simulink model "ARDronePFC"  (R2023b)
settings: Solver=ode1  StartTime=0.0  StopTime=200  FixedStep=simDT  RelTol=1e-3  EnableMultiTasking=on
values from neighbouring files (symbols this model uses):
  timeDelay = FMS.Ts*4    [setupEPFC.m]    (also in setupPFC.m)
undefined symbols (not defined in the file or in its folder): ssH, ssPitch, ssPitch2U, ssRoll, ssRoll2V, ssYaw
libraries: ARBlocks x3

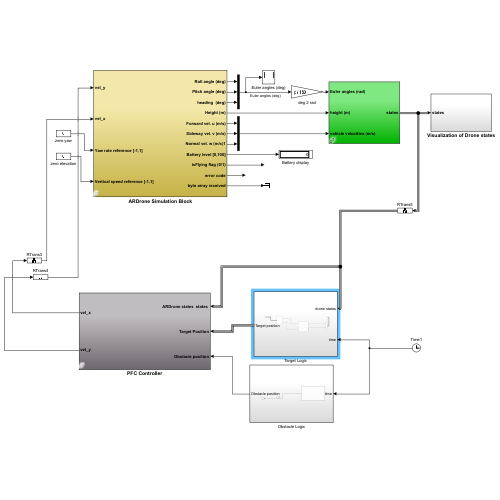
[thumbnail: Simulink's stored preview of the top-level diagram]
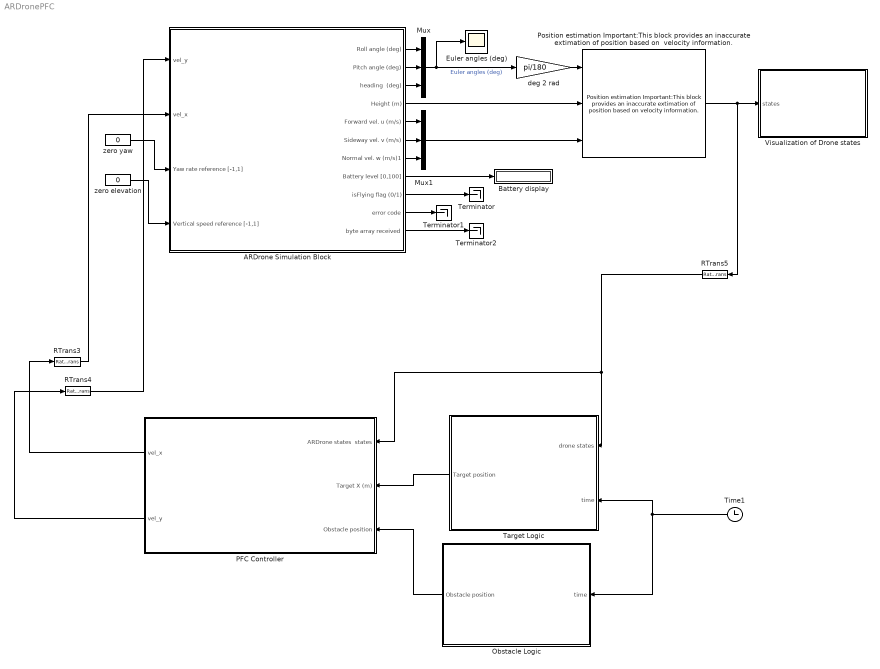
== system ARDronePFC ==
  ARDrone Simulation Block : Subsystem  AncestorBlock=ARBlocks/ARDrone Simulation Block
  Battery display : Display
  Euler angles (deg) : Scope
  Mux : Mux  Inputs=3
  Mux1 : Mux  Inputs=3
  Obstacle Logic : Subsystem
  PFC Controller : Subsystem  AncestorBlock=ARBlocks/Baseline Controller
  "Position estimation Important:This block provides an inaccurate extimation of position based on  velocity information. " : ARBlocks/Position estimation Important:This block provides an  inaccurate extimation of position  based on  velocity information.   SystemSampleTime=-1  VariantActivationTime=update diagram  AllowFlexibleInterface=on  Latency=0  AutoFrameSizeCalculation=off
  RTrans3 : RateTransition  OutPortSampleTime=simDT
  RTrans4 : RateTransition  OutPortSampleTime=simDT
  RTrans5 : RateTransition  OutPortSampleTime=FMS.Ts
  Target Logic : Subsystem
  Terminator : Terminator
  Terminator1 : Terminator
  Terminator2 : Terminator
  Time1 : Clock
  Visualization of Drone states : Subsystem
  deg 2 rad : Gain  Gain=pi/180
  zero elevation : Constant  Value=0
  zero yaw : Constant  Value=0
  wires:
  ARDrone Simulation Block/1(Roll angle (deg)) -> Mux/1
  ARDrone Simulation Block/2(Pitch angle (deg)) -> Mux/2
  ARDrone Simulation Block/5(Forward vel. u (m/s)) -> Mux1/1
  ARDrone Simulation Block/6(Sideway vel. v (m/s)) -> Mux1/2
  ARDrone Simulation Block/7(Normal vel. w (m/s)1) -> Mux1/3
  Mux/1 -> deg 2 rad/1, Euler angles (deg)/1  "Euler angles (deg)"
  ARDrone Simulation Block/8(Battery level [0,100]) -> Battery display/1
  PFC Controller/1(vel_x) -> RTrans3/1
  "Position estimation Important:This block provides an inaccurate extimation of position based on  velocity information. "/1 -> RTrans5/1, Visualization of Drone states/1(states)
  deg 2 rad/1 -> "Position estimation Important:This block provides an inaccurate extimation of position based on  velocity information. "/1
  ARDrone Simulation Block/4(Height (m)) -> "Position estimation Important:This block provides an inaccurate extimation of position based on  velocity information. "/2
  Mux1/1 -> "Position estimation Important:This block provides an inaccurate extimation of position based on  velocity information. "/3
  PFC Controller/2(vel_y) -> RTrans4/1
  ARDrone Simulation Block/3(heading  (deg)) -> Mux/3
  ARDrone Simulation Block/9(isFlying flag (0/1)) -> Terminator/1
  RTrans3/1 -> ARDrone Simulation Block/2(vel_x)
  RTrans4/1 -> ARDrone Simulation Block/1(vel_y)
  ARDrone Simulation Block/10(error code) -> Terminator1/1
  ARDrone Simulation Block/11(byte array received) -> Terminator2/1
  RTrans5/1 -> Target Logic/1(drone states), PFC Controller/1("ARDrone states  states ")
  zero yaw/1 -> ARDrone Simulation Block/3(Yaw rate reference [-1,1])
  zero elevation/1 -> ARDrone Simulation Block/4(Vertical speed reference [-1,1])
  Target Logic/1(Target position) -> PFC Controller/2(Target X (m))
  Obstacle Logic/1(Obstacle position) -> PFC Controller/3(Obstacle position)
  Time1/1 -> Target Logic/2(time), Obstacle Logic/1(time)

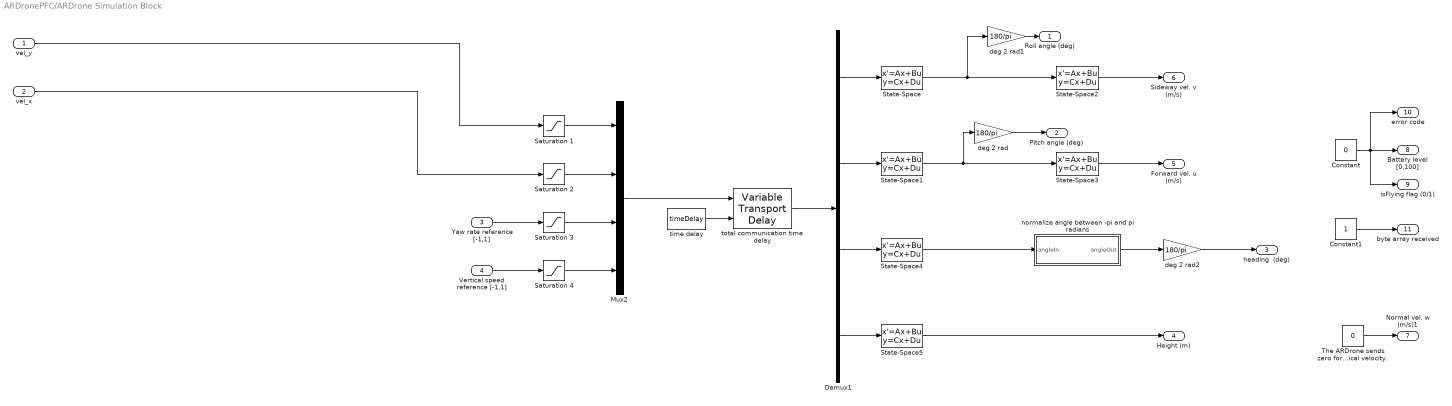
== system ARDronePFC/ARDrone Simulation Block ==
  vel_y : Inport
  vel_x : Inport  Port=2
  Yaw rate reference [-1,1] : Inport  Port=3
  Vertical speed reference [-1,1] : Inport  Port=4
  Constant : Constant  Value=0
  Constant1 : Constant
  Demux1 : Demux
  Mux2 : Mux
  Saturation {1..4} (4 alike) : Saturate  UpperLimit=1  LowerLimit=-1
  State-Space : StateSpace  A=ssRoll.a  B=ssRoll.b  C=ssRoll.c  D=ssRoll.d  InitialCondition=0
  State-Space1 : StateSpace  A=ssPitch.a  B=ssPitch.b  C=ssPitch.c  D=ssPitch.d  InitialCondition=0
  State-Space2 : StateSpace  A=ssRoll2V.a  B=ssRoll2V.b  C=ssRoll2V.c  D=ssRoll2V.d  InitialCondition=0
  State-Space3 : StateSpace  A=ssPitch2U.a  B=ssPitch2U.b  C=ssPitch2U.c  D=ssPitch2U.d  InitialCondition=0
  State-Space4 : StateSpace  A=ssYaw.a  B=ssYaw.b  C=ssYaw.c  D=ssYaw.d  InitialCondition=0
  State-Space5 : StateSpace  A=ssH.a  B=ssH.b  C=ssH.c  D=ssH.d  InitialCondition=0
  "The ARDrone sends zero for the vertical velocity. " : Constant  Value=0
  deg 2 rad : Gain  Gain=180/pi
  deg 2 rad1 : Gain  Gain=180/pi
  deg 2 rad2 : Gain  Gain=180/pi
  normalize angle between -pi and pi radians : MATLAB Function  TreatAsAtomicUnit=on
  time delay : Constant  Value=timeDelay
  total communication time delay : VariableTransportDelay  MaximumDelay=10  InitialOutput=[0 0 0 0]  MaximumPoints=4096
  Roll angle (deg) : Outport
  Pitch angle (deg) : Outport  Port=2
  heading  (deg) : Outport  Port=3
  Height (m) : Outport  Port=4
  Forward vel. u (m/s) : Outport  Port=5
  Sideway vel. v (m/s) : Outport  Port=6
  Normal vel. w (m/s)1 : Outport  Port=7
  Battery level [0,100] : Outport  Port=8
  isFlying flag (0/1) : Outport  Port=9
  error code : Outport  Port=10
  byte array received : Outport  Port=11
  wires:
  "The ARDrone sends zero for the vertical velocity. "/1 -> Normal vel. w (m/s)1/1
  Constant1/1 -> byte array received/1
  deg 2 rad2/1 -> heading  (deg)/1
  deg 2 rad1/1 -> Roll angle (deg)/1
  deg 2 rad/1 -> Pitch angle (deg)/1
  Constant/1 -> Battery level [0,100]/1, error code/1, isFlying flag (0/1)/1
  normalize angle between -pi and pi radians/1(angleOut) -> deg 2 rad2/1
  State-Space5/1 -> Height (m)/1
  State-Space3/1 -> Forward vel. u (m/s)/1
  State-Space2/1 -> Sideway vel. v (m/s)/1
  State-Space4/1 -> normalize angle between -pi and pi radians/1(angleIn)
  Demux1/3 -> State-Space4/1
  Demux1/2 -> State-Space1/1
  Saturation 4/1 -> Mux2/4
  Saturation 3/1 -> Mux2/3
  Saturation 2/1 -> Mux2/2
  Saturation 1/1 -> Mux2/1
  total communication time delay/1 -> Demux1/1
  Mux2/1 -> total communication time delay/1
  time delay/1 -> total communication time delay/2
  State-Space1/1 -> State-Space3/1, deg 2 rad/1
  State-Space/1 -> State-Space2/1, deg 2 rad1/1
  Demux1/4 -> State-Space5/1
  Demux1/1 -> State-Space/1
  Vertical speed reference [-1,1]/1 -> Saturation 4/1
  Yaw rate reference [-1,1]/1 -> Saturation 3/1
  vel_x/1 -> Saturation 2/1
  vel_y/1 -> Saturation 1/1

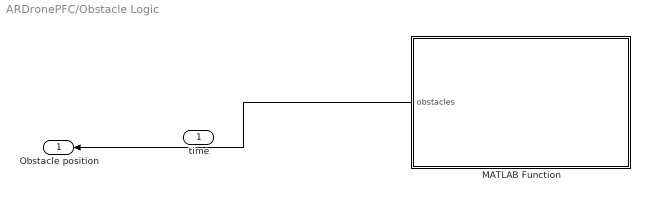
== system ARDronePFC/Obstacle Logic ==
  time : Inport
  MATLAB Function : MATLAB Function  TreatAsAtomicUnit=on
  Obstacle position : Outport
  wires:
  MATLAB Function/1(obstacles) -> Obstacle position/1

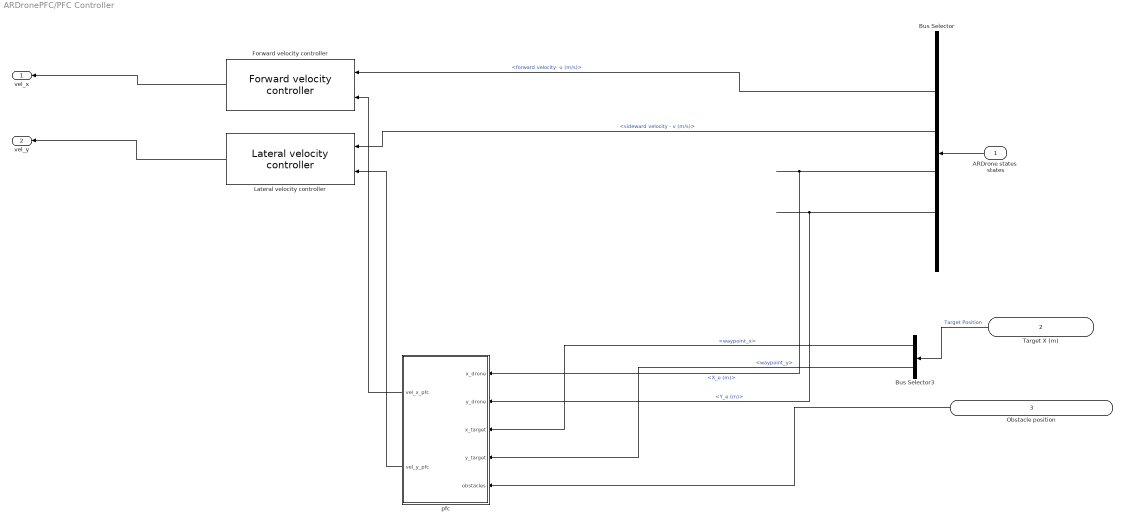
== system ARDronePFC/PFC Controller ==
  "ARDrone states  states " : Inport
  Target X (m) : Inport  Port=2
  Obstacle position : Inport  Port=3
  Bus Selector : BusSelector  OutputSignals=h (m),forward velocity- u (m/s),sideward velocity - v (m/s),X_e (m),Y_e (m),yaw angle (rad)
  Bus Selector3 : BusSelector  OutputSignals=waypoint_x,waypoint_y
  "Forward velocity controller " : ARBlocks/Baseline Controller/Forward velocity controller   SystemSampleTime=-1  VariantActivationTime=update diagram  AllowFlexibleInterface=on  Latency=0  AutoFrameSizeCalculation=off
  Lateral velocity controller : ARBlocks/Baseline Controller/Lateral velocity controller  SystemSampleTime=-1  VariantActivationTime=update diagram  AllowFlexibleInterface=on  Latency=0  AutoFrameSizeCalculation=off
  pfc : MATLAB Function  TreatAsAtomicUnit=on
  vel_x : Outport
  vel_y : Outport  Port=2
  wires:
  Bus Selector/3 -> Lateral velocity controller/1  "<sideward velocity - v (m/s)>"
  Bus Selector/5 -> pfc/2(y_drone)  "<Y_e (m)>"
  Bus Selector/4 -> pfc/1(x_drone)  "<X_e (m)>"
  Bus Selector/2 -> "Forward velocity controller "/1  "<forward velocity- u (m/s)>"
  "ARDrone states  states "/1 -> Bus Selector/1
  pfc/1(vel_x_pfc) -> "Forward velocity controller "/2
  pfc/2(vel_y_pfc) -> Lateral velocity controller/2
  "Forward velocity controller "/1 -> vel_x/1
  Lateral velocity controller/1 -> vel_y/1
  Target X (m)/1 -> Bus Selector3/1  "Target Position"
  Bus Selector3/1 -> pfc/3(x_target)  "<waypoint_x>"
  Bus Selector3/2 -> pfc/4(y_target)  "<waypoint_y>"
  Obstacle position/1 -> pfc/5(obstacles)

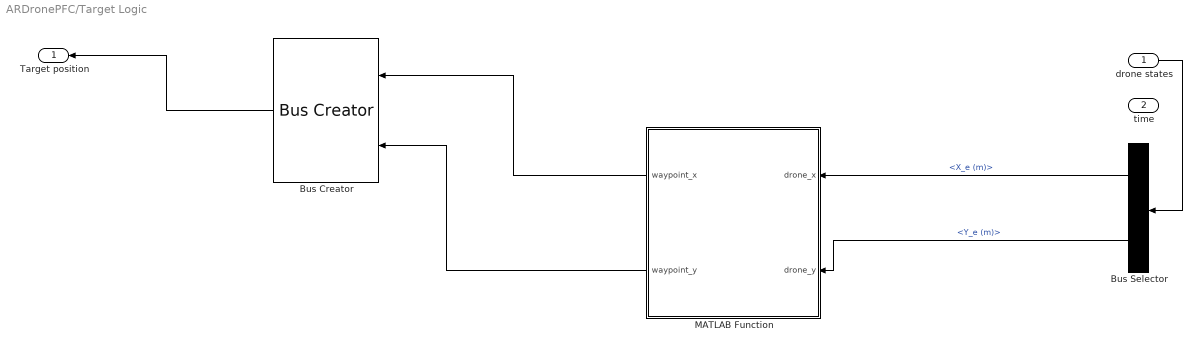
== system ARDronePFC/Target Logic ==
  drone states : Inport
  time : Inport  Port=2
  Bus Creator : BusCreator  Inputs=2
  Bus Selector : BusSelector  OutputSignals=X_e (m),Y_e (m)
  MATLAB Function : MATLAB Function  TreatAsAtomicUnit=on
  Target position : Outport
  wires:
  Bus Creator/1 -> Target position/1
  drone states/1 -> Bus Selector/1
  Bus Selector/1 -> MATLAB Function/1(drone_x)  "<X_e (m)>"
  Bus Selector/2 -> MATLAB Function/2(drone_y)  "<Y_e (m)>"
  MATLAB Function/1(waypoint_x) -> Bus Creator/1
  MATLAB Function/2(waypoint_y) -> Bus Creator/2

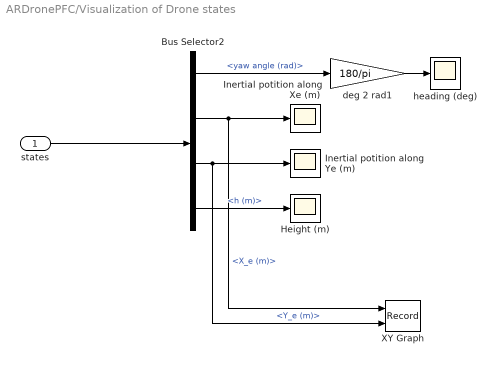
== system ARDronePFC/Visualization of Drone states ==
  states : Inport
  Bus Selector2 : BusSelector  OutputSignals=yaw angle (rad),X_e (m),Y_e (m),h (m)
  Height (m) : Scope
  Inertial potition along Xe (m) : Scope
  Inertial potition along Ye (m) : Scope
  XY Graph : Record  FileSettingsInternal="{\"entries\":[{\"content\":{\"excelSettings\":{\"content\":{},\"type\":\"Streamout.ExcelSettings\"}},\"type\":\"Streamout.FileSettingStorage\",\"uuid\":\"\"}],\"packageUris\":[\"http:\\/\\/schema.mathworks.com\\/mf0\\/streamout_blocks\\/R2020a\"],\"version\":\"1.0\"}"  Layout=[1 1]  SignalsInternal="{\"entries\":[{\"content\":{\"signals\":[{\"content\":{\"blockPath\":[],\"dimensions\":[1],\"domain\":\"\",\"lineColor\":\"#a2142f\",\"plots\":[1],\"port\":1,\"sid\":[\"\"],\"signalID\":805,\"signalName\":\"<X_e (m)>\"},\"type\":\"RecordBlkView.Signal\",\"uuid\":\"\"},{\"content\":{\"blockPath\":[],\"dimensions\":[1],\"domain\":\"\",\"lineColor\":\"#139fff\",\"plots\":[1],\"port\":2,\"sid\":[\"\"],\"signalID\":809,\"signalName\":\"<Y_e (m)>\"},\"type\":\"RecordBlkView. ...(+164 chars)"  VisualizationBindings="{\"xyplotplugin\":{\"info\":[{\"series\":[{\"bindingParametersList\":[{\"parameter\":\"Y-Axis\",\"signalID\":809,\"signalName\":\"<Y_e (m)>\"},{\"parameter\":\"X-Axis\",\"signalID\":805,\"signalName\":\"<X_e (m)>\"}],\"seriesID\":33325}],\"subplotID\":1}]}}"  CompatibilityTag=XY
  deg 2 rad1 : Gain  Gain=180/pi
  heading (deg) : Scope
  wires:
  states/1 -> Bus Selector2/1
  Bus Selector2/1 -> deg 2 rad1/1  "<yaw angle (rad)>"
  Bus Selector2/2 -> XY Graph/1, Inertial potition along Xe (m)/1  "<X_e (m)>"
  Bus Selector2/3 -> XY Graph/2, Inertial potition along Ye (m)/1  "<Y_e (m)>"
  Bus Selector2/4 -> Height (m)/1  "<h (m)>"
  deg 2 rad1/1 -> heading (deg)/1

== matlab function ARDronePFC/Target Logic/MATLAB Function ==
function [waypoint_x, waypoint_y] = fcn(drone_x, drone_y)

%Define waypoints

waypoint_1 = [2.5 -1];
waypoint_2 = [2.5 1]; 
waypoint_3 = [-2.5 1];
waypoint_4 = [-2.5 -1];
waypoint_5 = [2.5  -1];

waypoint =[waypoint_1; waypoint_2;waypoint_3 ; waypoint_4; waypoint_5  ];
number_of_WayPoints = 5;
         
persistent waypointPTR;

if isempty(waypointPTR)
    waypointPTR = 1;
end


% We assume  drone has reached waypoint if distance between waypoint and
% drone is less than 0.1m. We then set the next waypoint as target.

if ( norm([drone_x drone_y] - waypoint( waypointPTR,:) )< 0.1)
    
    if(waypointPTR ~= number_of_WayPoints)
                 if(waypointPTR < number_of_WayPoints)
                    waypointPTR = waypointPTR+ 1
                  
                 end           
    end

end

wp = waypoint(waypointPTR,:)
waypoint_x = wp(1);
waypoint_y = wp(2);

== matlab function ARDronePFC/PFC Controller/pfc ==
function [vel_x_pfc, vel_y_pfc]= pfc(x_drone, y_drone, x_target, y_target, obstacles)

lamda_one = 0.2;

pos_drone = [x_drone y_drone];
pos_target = [x_target y_target];

vel_attraction = -lamda_one.*(pos_drone - pos_target);

etha_one = 0.03;
obs_range = 1.0;
vel_repulsion = [0 0];

for obs = 1:size(obstacles, 1)

if norm(pos_drone - obstacles(obs,:)) <= obs_range
    vel_repulsion = vel_repulsion + (pos_drone - obstacles(obs,:)).*(etha_one/(norm(pos_drone - obstacles(obs,:))^4));
   
end
end

vel_pfc = vel_attraction + vel_repulsion;

vel_x_pfc = vel_pfc(1);
vel_y_pfc = vel_pfc(2);

== matlab function ARDronePFC/Obstacle Logic/MATLAB Function ==
function obstacles  = fcn

obstacle_1 = [1 1];



obstacles = [obstacle_1]

== matlab function ARDronePFC/ARDrone Simulation Block/normalize angle between -pi and pi radians ==
function angleOut = fcn(angleIn)
%#codegen

angleOut = mod(angleIn, 2*pi) ;
if angleOut > pi
    angleOut = -2*pi + angleOut ; 
end
